simulink model "HANcoder_E407_TTA_Controller_v2"  (R2018b)
settings: Solver=FixedStepDiscrete  StartTime=0.0  StopTime=1  FixedStep=0.01  RelTol=1e-3
PreLoadFcn:
  | librarySetup
  | eval([bdroot,'_startup']) %Calling [modelName]_startup.m
values from neighbouring files (symbols this model uses):
  basic_cycle_duration_bc0 = TM_Reset_Board   + COMP_duration    (= 212)    [HANcoder_E407_TTA_Controller_v3_startup.m]
  basic_cycle_duration_bc1 = TM_Reset_Var_bc1 + COMP_duration    (= 288)    [HANcoder_E407_TTA_Controller_v3_startup.m]
  comm_delay_estimation1 = round(comm_delay_measured1*hardware_granularity/frequency_IRQ)    [HANcoder_E407_TTA_Controller_v3_startup.m]
  comm_delay_estimation2 = round(comm_delay_measured2*hardware_granularity/frequency_IRQ)    [HANcoder_E407_TTA_Controller_v3_startup.m]
  COMM_Period = 40    [HANcoder_E407_TTA_Controller_v3_startup.m]
  COMM_Phase1 = Simulink.Parameter    [HANcoder_E407_TTA_Controller_v3_startup.m]
  COMM_Phase2 = Simulink.Parameter    [HANcoder_E407_TTA_Controller_v3_startup.m]
  COMP_duration = 4    [HANcoder_E407_TTA_Controller_v3_startup.m]
  Controller1_Board = 1    [HANcoder_E407_TTA_Controller_v3_startup.m]
  Controller2_Board = 2    [HANcoder_E407_TTA_Controller_v3_startup.m]
  Controller3_Board = 3    [HANcoder_E407_TTA_Controller_v3_startup.m]
  delta_max = 1    [HANcoder_E407_TTA_Controller_v3_startup.m]
  delta_min = -1    [HANcoder_E407_TTA_Controller_v3_startup.m]
  delta_precision = 6    [HANcoder_E407_TTA_Controller_v3_startup.m]
  e_width = 0.1    [HANcoder_E407_TTA_Controller_v3_startup.m]
  frequency_IRQ = 100    [HANcoder_E407_TTA_Controller_v3_startup.m]
  HANtuneOverride = Simulink.Parameter    [HANcoder_E407_TTA_Controller_v3_startup.m]
  hardware_granularity = 1000000    [HANcoder_E407_TTA_Controller_v3_startup.m]
  I_a = 2.25    [HANcoder_E407_TTA_Controller_v3_startup.m]
  I_f = 2.25    [HANcoder_E407_TTA_Controller_v3_startup.m]
  idle_time_init = basic_cycle_duration_bc0 + basic_cycle_duration_bc1    (= 500)    [HANcoder_E407_TTA_Controller_v3_startup.m]
  Input_Gen_Board = 4    [HANcoder_E407_TTA_Controller_v3_startup.m]
  LA_Clock_Gr = 1    [HANcoder_E407_TTA_Controller_v3_startup.m]
  LA_COMM_Err = 1    [HANcoder_E407_TTA_Controller_v3_startup.m]
  LA_MEX_Flag = 1    [HANcoder_E407_TTA_Controller_v3_startup.m]
  LA_Task_Act = 1    [HANcoder_E407_TTA_Controller_v3_startup.m]
  m_v = 100.0    (= 100)    [HANcoder_E407_TTA_Controller_v3_startup.m]
  Master_Role = 1    [HANcoder_E407_TTA_Controller_v3_startup.m]
  matrix_cycle_duration = basic_cycle_duration_bc0 + basic_cycle_duration_bc1    (= 500)    [HANcoder_E407_TTA_Controller_v3_startup.m]
  matrix_rows = 2    [HANcoder_E407_TTA_Controller_v3_startup.m]
  max_num_msgs_CAN1 = 2^Tx_bit_number-1    (= 7)    [HANcoder_E407_TTA_Controller_v3_startup.m]
  max_num_msgs_CAN2 = max_num_msgs_CAN1    (= 7)    [HANcoder_E407_TTA_Controller_v3_startup.m]
  OutControl1_ID = 23    [HANcoder_E407_TTA_Controller_v3_startup.m]
  OutControl2_ID = 24    [HANcoder_E407_TTA_Controller_v3_startup.m]
  OutEmulator_ID = 25    [HANcoder_E407_TTA_Controller_v3_startup.m]
  R_al = 0.10    (= 0.1)    [HANcoder_E407_TTA_Controller_v3_startup.m]
  R_ar = 0.10    (= 0.1)    [HANcoder_E407_TTA_Controller_v3_startup.m]
  R_fl = 0.10    (= 0.1)    [HANcoder_E407_TTA_Controller_v3_startup.m]
  R_fr = 0.10    (= 0.1)    [HANcoder_E407_TTA_Controller_v3_startup.m]
  SensorValues_ID = 22    [HANcoder_E407_TTA_Controller_v3_startup.m]
  SetValues_ID = 21    [HANcoder_E407_TTA_Controller_v3_startup.m]
  Slave_Role = 2    [HANcoder_E407_TTA_Controller_v3_startup.m]
  speed_k_d = Simulink.Parameter    [HANcoder_E407_TTA_Controller_v3_startup.m]
  speed_k_i = Simulink.Parameter    [HANcoder_E407_TTA_Controller_v3_startup.m]
  speed_k_p = Simulink.Parameter    [HANcoder_E407_TTA_Controller_v3_startup.m]
  speed_max = 10    [HANcoder_E407_TTA_Controller_v3_startup.m]
  speed_min = -10    [HANcoder_E407_TTA_Controller_v3_startup.m]
  speed_precision = 3    [HANcoder_E407_TTA_Controller_v3_startup.m]
  Sync_ID = 1    [HANcoder_E407_TTA_Controller_v3_startup.m]
  tau_max = 5    [HANcoder_E407_TTA_Controller_v3_startup.m]
  tau_min = -5    [HANcoder_E407_TTA_Controller_v3_startup.m]
  tau_range = abs(tau_max) + abs(tau_min)    [HANcoder_E407_TTA_Controller_v3_startup.m]
  theta_max = (speed_max/R_fr)*matrix_cycle_duration*frequency_IRQ/hardware_granularity    (= 5)    [HANcoder_E407_TTA_Controller_v3_startup.m]
  theta_min = (-1)*theta_max    (= -5)    [HANcoder_E407_TTA_Controller_v3_startup.m]
  theta_precision = 7-(fix(log2(theta_max))+1)    [HANcoder_E407_TTA_Controller_v3_startup.m]
  Tl_a = 0.6    [HANcoder_E407_TTA_Controller_v3_startup.m]
  Tl_f = 0.6    [HANcoder_E407_TTA_Controller_v3_startup.m]
  TM_Check_Output_Control1 = TM_COMM_Output_Control1 + COMM_duration    (= 188)    [HANcoder_E407_TTA_Controller_v3_startup.m]
  TM_Check_Output_Control2 = TM_COMM_Output_Control2 + COMM_duration    (= 232)    [HANcoder_E407_TTA_Controller_v3_startup.m]
  TM_Check_Output_Emulator = TM_COMM_Output_Emulator + COMM_duration    (= 280)    [HANcoder_E407_TTA_Controller_v3_startup.m]
  TM_Check_Sensor_Values = TM_COMM_Sensor_Values + COMM_duration    (= 132)    [HANcoder_E407_TTA_Controller_v3_startup.m]
  TM_Check_Set_Values = TM_COMM_Set_Values + COMM_duration    (= 88)    [HANcoder_E407_TTA_Controller_v3_startup.m]
  TM_Check_Sync = TM_COMM_Sync   + COMM_duration    (= 40)    [HANcoder_E407_TTA_Controller_v3_startup.m]
  TM_Check_TOuts = TM_Count_Vote3 + COMP_duration    (= 196)    [HANcoder_E407_TTA_Controller_v3_startup.m]
  TM_Check_Vote1 = TM_COMM_Vote1  + COMM_duration    (= 92)    [HANcoder_E407_TTA_Controller_v3_startup.m]
  TM_Check_Vote2 = TM_COMM_Vote2  + COMM_duration    (= 140)    [HANcoder_E407_TTA_Controller_v3_startup.m]
  TM_Check_Vote3 = TM_COMM_Vote3  + COMM_duration    (= 188)    [HANcoder_E407_TTA_Controller_v3_startup.m]
  TM_COMM_Output_Control1 = TM_Velocity + COMP_duration    (= 148)    [HANcoder_E407_TTA_Controller_v3_startup.m]
  TM_COMM_Output_Control2 = TM_Check_Output_Control1 + COMP_duration    (= 192)    [HANcoder_E407_TTA_Controller_v3_startup.m]
  TM_COMM_Output_Emulator = TM_TMR + COMP_duration    (= 240)    [HANcoder_E407_TTA_Controller_v3_startup.m]
  TM_COMM_Sensor_Values = TM_Check_Set_Values + COMP_duration    (= 92)    [HANcoder_E407_TTA_Controller_v3_startup.m]
  TM_COMM_Set_Values = TM_Update_LT + COMP_duration    (= 48)    [HANcoder_E407_TTA_Controller_v3_startup.m]
  TM_COMM_Sync = basic_cycle_start    (= 0)    [HANcoder_E407_TTA_Controller_v3_startup.m]
  TM_COMM_Vote1 = TM_Vote_Dec    + COMP_duration    (= 52)    [HANcoder_E407_TTA_Controller_v3_startup.m]
  TM_COMM_Vote2 = TM_Count_Vote1 + COMP_duration    (= 100)    [HANcoder_E407_TTA_Controller_v3_startup.m]
  TM_COMM_Vote3 = TM_Count_Vote2 + COMP_duration    (= 148)    [HANcoder_E407_TTA_Controller_v3_startup.m]
  TM_Count_Vote1 = TM_Check_Vote1 + COMP_duration    (= 96)    [HANcoder_E407_TTA_Controller_v3_startup.m]
  TM_Count_Vote2 = TM_Check_Vote2 + COMP_duration    (= 144)    [HANcoder_E407_TTA_Controller_v3_startup.m]
  TM_Count_Vote3 = TM_Check_Vote3 + COMP_duration    (= 192)    [HANcoder_E407_TTA_Controller_v3_startup.m]
  TM_Data_bc0 = TM_COMM_Sync    (= 0)    [HANcoder_E407_TTA_Controller_v3_startup.m]
  TM_Data_bc1 = TM_Data_bc0(1:4)    [HANcoder_E407_TTA_Controller_v3_startup.m]
  TM_New_Master = TM_Check_TOuts + COMP_duration    (= 200)    [HANcoder_E407_TTA_Controller_v3_startup.m]
  TM_Reset_Board = TM_Reset_Var   + COMP_duration    (= 208)    [HANcoder_E407_TTA_Controller_v3_startup.m]
  TM_Reset_Var = TM_New_Master  + COMP_duration    (= 204)    [HANcoder_E407_TTA_Controller_v3_startup.m]
  TM_Reset_Var_bc1 = TM_Check_Output_Emulator + COMP_duration    (= 284)    [HANcoder_E407_TTA_Controller_v3_startup.m]
  TM_Steer = TM_Check_Sensor_Values + COMP_duration    (= 136)    [HANcoder_E407_TTA_Controller_v3_startup.m]
  TM_TMR = TM_Check_Output_Control2 + COMP_duration    (= 236)    [HANcoder_E407_TTA_Controller_v3_startup.m]
  TM_Torque = TM_Steer + COMP_duration    (= 140)    [HANcoder_E407_TTA_Controller_v3_startup.m]
  TM_Type_bc0 = COMM    (= 0)    [HANcoder_E407_TTA_Controller_v3_startup.m]
  TM_Type_bc1 = TM_Type_bc0(1:4)    [HANcoder_E407_TTA_Controller_v3_startup.m]
  TM_Update_LT = TM_Check_Sync  + COMP_duration    (= 44)    [HANcoder_E407_TTA_Controller_v3_startup.m]
  TM_Velocity = TM_Torque + COMP_duration    (= 144)    [HANcoder_E407_TTA_Controller_v3_startup.m]
  TM_Vote_Dec = TM_Update_LT   + COMP_duration    (= 48)    [HANcoder_E407_TTA_Controller_v3_startup.m]
  torque_a_k_d = Simulink.Parameter    [HANcoder_E407_TTA_Controller_v3_startup.m]
  torque_a_k_i = Simulink.Parameter    [HANcoder_E407_TTA_Controller_v3_startup.m]
  torque_a_k_p = Simulink.Parameter    [HANcoder_E407_TTA_Controller_v3_startup.m]
  torque_f_k_d = Simulink.Parameter    [HANcoder_E407_TTA_Controller_v3_startup.m]
  torque_f_k_i = Simulink.Parameter    [HANcoder_E407_TTA_Controller_v3_startup.m]
  torque_f_k_p = Simulink.Parameter    [HANcoder_E407_TTA_Controller_v3_startup.m]
  torque_precision = 4    [HANcoder_E407_TTA_Controller_v3_startup.m]
  Vehicle_Em_Board = 5    [HANcoder_E407_TTA_Controller_v3_startup.m]
  Vote1_ID = 11    [HANcoder_E407_TTA_Controller_v3_startup.m]
  Vote2_ID = 12    [HANcoder_E407_TTA_Controller_v3_startup.m]
  Vote3_ID = 13    [HANcoder_E407_TTA_Controller_v3_startup.m]
undefined symbols (not defined in the file or in its folder): A0, A1, A2, A3, A4, CON2
libraries: hdlsllib x235, HANcoder_STM32_Target x25, simulink x3, simulink_extras x1
(part 21 of 22)

== system HANcoder_E407_TTA_Controller_v2/HANcoder STM32 Target - E407-STM32 algorithm/Global Ticks Increment/CAN Management/Matrix Cycle Manager/Subsystem/controller basic cycle 1/COMP Task - Rx_Output_Control2_Check/Process_Messages/Demux message CAN1 and check coherence1/msg_count>2_DEBUG ==
  note: If this board received during this COMM a message
      | with a count greater than 1, it means the first message
      | sent was missed, but at least one later msg reached
      | this board.
  msg_c : Inport
  Constant : Constant
  Constant1 : Constant
  Data Store Read : DataStoreRead  DataStoreName=msg_count_DEBUG
  Data Store Read1 : DataStoreRead  DataStoreName=msg_count_DEBUG
  Data Store Write : DataStoreWrite  DataStoreName=msg_count_DEBUG
  GreaterThan : RelationalOperator  Operator=>  OutDataTypeStr=boolean  RndMeth=Simplest
  Plus : Sum
  Switch : Switch  Criteria=u2 > Threshold
  wires:
  msg_c/1 -> GreaterThan/1
  Data Store Read/1 -> Switch/3
  Plus/1 -> Switch/1
  Data Store Read1/1 -> Plus/1
  Constant/1 -> Plus/2
  Switch/1 -> Data Store Write/1
  GreaterThan/1 -> Switch/2
  Constant1/1 -> GreaterThan/2

== system HANcoder_E407_TTA_Controller_v2/HANcoder STM32 Target - E407-STM32 algorithm/Global Ticks Increment/CAN Management/Matrix Cycle Manager/Subsystem/controller basic cycle 1/COMP Task - Rx_Output_Emulator_Check/Process_Messages/Demux message CAN1 and check coherence/Subsystem ==
  Msg_Temporal_Data : Inport
  Bit Shift : hdlsllib/Logic and Bit Operations/Bit Shift  mode=Shift Right Logical  N=7
      settings: SourceProductName=HDL Coder  SourceProductBaseCode=HD
  Bit Shift1 : hdlsllib/Logic and Bit Operations/Bit Shift  mode=Shift Right Logical  N=5
      settings: SourceProductName=HDL Coder  SourceProductBaseCode=HD
  Bit Shift2 : hdlsllib/Logic and Bit Operations/Bit Shift  mode=Shift Right Logical  N=4
      settings: SourceProductName=HDL Coder  SourceProductBaseCode=HD
  Bit Shift3 : hdlsllib/Logic and Bit Operations/Bit Shift  mode=Shift Left Logical  N=1
      settings: SourceProductName=HDL Coder  SourceProductBaseCode=HD
  Bit Shift4 : hdlsllib/Logic and Bit Operations/Bit Shift  mode=Shift Left Logical  N=4
      settings: SourceProductName=HDL Coder  SourceProductBaseCode=HD
  basic_cycle : Outport
  msg_count : Outport  Port=2
  board_id : Outport  Port=3
  wires:
  Bit Shift2/1 -> board_id/1
  Bit Shift/1 -> basic_cycle/1
  Msg_Temporal_Data/1 -> Bit Shift3/1, Bit Shift/1, Bit Shift4/1
  Bit Shift3/1 -> Bit Shift1/1
  Bit Shift1/1 -> msg_count/1
  Bit Shift4/1 -> Bit Shift2/1

== system HANcoder_E407_TTA_Controller_v2/HANcoder STM32 Target - E407-STM32 algorithm/Global Ticks Increment/CAN Management/Matrix Cycle Manager/Subsystem/controller basic cycle 1/COMP Task - Rx_Output_Emulator_Check/Process_Messages/Demux message CAN1 and check coherence/msg_count>2_DEBUG ==
  note: If this board received during this COMM a message
      | with a count greater than 1, it means the first message
      | sent was missed, but at least one later msg reached
      | this board.
  msg_c : Inport
  Constant : Constant
  Constant1 : Constant
  Data Store Read : DataStoreRead  DataStoreName=msg_count_DEBUG
  Data Store Read1 : DataStoreRead  DataStoreName=msg_count_DEBUG
  Data Store Write : DataStoreWrite  DataStoreName=msg_count_DEBUG
  GreaterThan : RelationalOperator  Operator=>  OutDataTypeStr=boolean  RndMeth=Simplest
  Plus : Sum
  Switch : Switch  Criteria=u2 > Threshold
  wires:
  Constant1/1 -> GreaterThan/2
  GreaterThan/1 -> Switch/2
  Switch/1 -> Data Store Write/1
  Constant/1 -> Plus/2
  Data Store Read1/1 -> Plus/1
  Plus/1 -> Switch/1
  Data Store Read/1 -> Switch/3
  msg_c/1 -> GreaterThan/1

== system HANcoder_E407_TTA_Controller_v2/HANcoder STM32 Target - E407-STM32 algorithm/Global Ticks Increment/CAN Management/Matrix Cycle Manager/Subsystem/controller basic cycle 1/COMP Task - Rx_Output_Emulator_Check/Process_Messages/Demux message CAN1 and check coherence1/Subsystem ==
  Msg_Temporal_Data : Inport
  Bit Shift : hdlsllib/Logic and Bit Operations/Bit Shift  mode=Shift Right Logical  N=7
      settings: SourceProductName=HDL Coder  SourceProductBaseCode=HD
  Bit Shift1 : hdlsllib/Logic and Bit Operations/Bit Shift  mode=Shift Right Logical  N=5
      settings: SourceProductName=HDL Coder  SourceProductBaseCode=HD
  Bit Shift2 : hdlsllib/Logic and Bit Operations/Bit Shift  mode=Shift Right Logical  N=4
      settings: SourceProductName=HDL Coder  SourceProductBaseCode=HD
  Bit Shift3 : hdlsllib/Logic and Bit Operations/Bit Shift  mode=Shift Left Logical  N=1
      settings: SourceProductName=HDL Coder  SourceProductBaseCode=HD
  Bit Shift4 : hdlsllib/Logic and Bit Operations/Bit Shift  mode=Shift Left Logical  N=4
      settings: SourceProductName=HDL Coder  SourceProductBaseCode=HD
  basic_cycle : Outport
  msg_count : Outport  Port=2
  board_id : Outport  Port=3
  wires:
  Bit Shift4/1 -> Bit Shift2/1
  Bit Shift3/1 -> Bit Shift1/1
  Bit Shift2/1 -> board_id/1
  Bit Shift1/1 -> msg_count/1
  Msg_Temporal_Data/1 -> Bit Shift3/1, Bit Shift/1, Bit Shift4/1
  Bit Shift/1 -> basic_cycle/1

== system HANcoder_E407_TTA_Controller_v2/HANcoder STM32 Target - E407-STM32 algorithm/Global Ticks Increment/CAN Management/Matrix Cycle Manager/Subsystem/controller basic cycle 1/COMP Task - Rx_Output_Emulator_Check/Process_Messages/Demux message CAN1 and check coherence1/msg_count>2_DEBUG ==
  note: If this board received during this COMM a message
      | with a count greater than 1, it means the first message
      | sent was missed, but at least one later msg reached
      | this board.
  msg_c : Inport
  Constant : Constant
  Constant1 : Constant
  Data Store Read : DataStoreRead  DataStoreName=msg_count_DEBUG
  Data Store Read1 : DataStoreRead  DataStoreName=msg_count_DEBUG
  Data Store Write : DataStoreWrite  DataStoreName=msg_count_DEBUG
  GreaterThan : RelationalOperator  Operator=>  OutDataTypeStr=boolean  RndMeth=Simplest
  Plus : Sum
  Switch : Switch  Criteria=u2 > Threshold
  wires:
  Constant1/1 -> GreaterThan/2
  GreaterThan/1 -> Switch/2
  Switch/1 -> Data Store Write/1
  Constant/1 -> Plus/2
  Data Store Read1/1 -> Plus/1
  Plus/1 -> Switch/1
  Data Store Read/1 -> Switch/3
  msg_c/1 -> GreaterThan/1

== system HANcoder_E407_TTA_Controller_v2/HANcoder STM32 Target - E407-STM32 algorithm/Global Ticks Increment/CAN Management/Matrix Cycle Manager/Subsystem/controller basic cycle 1/COMP Task - Rx_Sensor_Values_Check/Process_Messages/Demux message CAN1 and check coherence/Subsystem ==
  Msg_Temporal_Data : Inport
  Bit Shift : hdlsllib/Logic and Bit Operations/Bit Shift  mode=Shift Right Logical  N=7
      settings: SourceProductName=HDL Coder  SourceProductBaseCode=HD
  Bit Shift1 : hdlsllib/Logic and Bit Operations/Bit Shift  mode=Shift Right Logical  N=5
      settings: SourceProductName=HDL Coder  SourceProductBaseCode=HD
  Bit Shift2 : hdlsllib/Logic and Bit Operations/Bit Shift  mode=Shift Right Logical  N=4
      settings: SourceProductName=HDL Coder  SourceProductBaseCode=HD
  Bit Shift3 : hdlsllib/Logic and Bit Operations/Bit Shift  mode=Shift Left Logical  N=1
      settings: SourceProductName=HDL Coder  SourceProductBaseCode=HD
  Bit Shift4 : hdlsllib/Logic and Bit Operations/Bit Shift  mode=Shift Left Logical  N=4
      settings: SourceProductName=HDL Coder  SourceProductBaseCode=HD
  basic_cycle : Outport
  msg_count : Outport  Port=2
  board_id : Outport  Port=3
  wires:
  Bit Shift4/1 -> Bit Shift2/1
  Bit Shift1/1 -> msg_count/1
  Bit Shift3/1 -> Bit Shift1/1
  Msg_Temporal_Data/1 -> Bit Shift4/1, Bit Shift/1, Bit Shift3/1
  Bit Shift/1 -> basic_cycle/1
  Bit Shift2/1 -> board_id/1

== system HANcoder_E407_TTA_Controller_v2/HANcoder STM32 Target - E407-STM32 algorithm/Global Ticks Increment/CAN Management/Matrix Cycle Manager/Subsystem/controller basic cycle 1/COMP Task - Rx_Sensor_Values_Check/Process_Messages/Demux message CAN1 and check coherence/msg_count>2_DEBUG ==
  note: If this board received during this COMM a message
      | with a count greater than 1, it means the first message
      | sent was missed, but at least one later msg reached
      | this board.
  msg_c : Inport
  Constant : Constant
  Constant1 : Constant
  Data Store Read : DataStoreRead  DataStoreName=msg_count_DEBUG
  Data Store Read1 : DataStoreRead  DataStoreName=msg_count_DEBUG
  Data Store Write : DataStoreWrite  DataStoreName=msg_count_DEBUG
  GreaterThan : RelationalOperator  Operator=>  OutDataTypeStr=boolean  RndMeth=Simplest
  Plus : Sum
  Switch : Switch  Criteria=u2 > Threshold
  wires:
  msg_c/1 -> GreaterThan/1
  Data Store Read/1 -> Switch/3
  Plus/1 -> Switch/1
  Data Store Read1/1 -> Plus/1
  Constant/1 -> Plus/2
  Switch/1 -> Data Store Write/1
  GreaterThan/1 -> Switch/2
  Constant1/1 -> GreaterThan/2

== system HANcoder_E407_TTA_Controller_v2/HANcoder STM32 Target - E407-STM32 algorithm/Global Ticks Increment/CAN Management/Matrix Cycle Manager/Subsystem/controller basic cycle 1/COMP Task - Rx_Sensor_Values_Check/Process_Messages/Demux message CAN1 and check coherence1/Subsystem ==
  Msg_Temporal_Data : Inport
  Bit Shift : hdlsllib/Logic and Bit Operations/Bit Shift  mode=Shift Right Logical  N=7
      settings: SourceProductName=HDL Coder  SourceProductBaseCode=HD
  Bit Shift1 : hdlsllib/Logic and Bit Operations/Bit Shift  mode=Shift Right Logical  N=5
      settings: SourceProductName=HDL Coder  SourceProductBaseCode=HD
  Bit Shift2 : hdlsllib/Logic and Bit Operations/Bit Shift  mode=Shift Right Logical  N=4
      settings: SourceProductName=HDL Coder  SourceProductBaseCode=HD
  Bit Shift3 : hdlsllib/Logic and Bit Operations/Bit Shift  mode=Shift Left Logical  N=1
      settings: SourceProductName=HDL Coder  SourceProductBaseCode=HD
  Bit Shift4 : hdlsllib/Logic and Bit Operations/Bit Shift  mode=Shift Left Logical  N=4
      settings: SourceProductName=HDL Coder  SourceProductBaseCode=HD
  basic_cycle : Outport
  msg_count : Outport  Port=2
  board_id : Outport  Port=3
  wires:
  Bit Shift/1 -> basic_cycle/1
  Msg_Temporal_Data/1 -> Bit Shift4/1, Bit Shift/1, Bit Shift3/1
  Bit Shift1/1 -> msg_count/1
  Bit Shift2/1 -> board_id/1
  Bit Shift3/1 -> Bit Shift1/1
  Bit Shift4/1 -> Bit Shift2/1

== system HANcoder_E407_TTA_Controller_v2/HANcoder STM32 Target - E407-STM32 algorithm/Global Ticks Increment/CAN Management/Matrix Cycle Manager/Subsystem/controller basic cycle 1/COMP Task - Rx_Sensor_Values_Check/Process_Messages/Demux message CAN1 and check coherence1/msg_count>2_DEBUG ==
  note: If this board received during this COMM a message
      | with a count greater than 1, it means the first message
      | sent was missed, but at least one later msg reached
      | this board.
  msg_c : Inport
  Constant : Constant
  Constant1 : Constant
  Data Store Read : DataStoreRead  DataStoreName=msg_count_DEBUG
  Data Store Read1 : DataStoreRead  DataStoreName=msg_count_DEBUG
  Data Store Write : DataStoreWrite  DataStoreName=msg_count_DEBUG
  GreaterThan : RelationalOperator  Operator=>  OutDataTypeStr=boolean  RndMeth=Simplest
  Plus : Sum
  Switch : Switch  Criteria=u2 > Threshold
  wires:
  msg_c/1 -> GreaterThan/1
  Data Store Read/1 -> Switch/3
  Plus/1 -> Switch/1
  Data Store Read1/1 -> Plus/1
  Constant/1 -> Plus/2
  Switch/1 -> Data Store Write/1
  GreaterThan/1 -> Switch/2
  Constant1/1 -> GreaterThan/2

== system HANcoder_E407_TTA_Controller_v2/HANcoder STM32 Target - E407-STM32 algorithm/Global Ticks Increment/CAN Management/Matrix Cycle Manager/Subsystem/controller basic cycle 1/COMP Task - Rx_Sensor_Values_Check/Update Msg buffer/Sensor Values Rx Update/Inputs Rx OK ==
  note: Matrix cycles since last input value
  note: Ticks to seconds conversion
  note: For derivatives and integrals it is important to keep
      | track of how much time has passed since the last
      | time we received a set or sensor value.
  Enable : EnablePort
  Constant : Constant  Value=matrix_cycle_duration
  Constant1 : Constant
  Data Store Read : DataStoreRead  DataStoreName=mc_counter
  Data Store Write : DataStoreWrite  Priority=1  DataStoreName=rx_data_incr_time
  Data Store Write1 : DataStoreWrite  Priority=2  DataStoreName=mc_counter
  Gain : Gain  Gain=frequency_IRQ/hardware_granularity
  Multiply : Product
  wires:
  Constant/1 -> Gain/1
  Gain/1 -> Multiply/1
  Data Store Read/1 -> Multiply/2
  Multiply/1 -> Data Store Write/1
  Constant1/1 -> Data Store Write1/1

== system HANcoder_E407_TTA_Controller_v2/HANcoder STM32 Target - E407-STM32 algorithm/Global Ticks Increment/CAN Management/Matrix Cycle Manager/Subsystem/controller basic cycle 1/COMP Task - Rx_Sensor_Values_Check/Update Msg buffer/Sensor Values Rx Update/Not enough inputs ==
  note: If no inputs received, no calculations are done.
      | Next time set and sensor values are received
      | it is important to keep track of how much time
      | has passed for derivatives and integrals.
  Enable : EnablePort
  Constant : Constant
  Data Store Read : DataStoreRead  DataStoreName=mc_counter
  Data Store Write1 : DataStoreWrite  DataStoreName=mc_counter
  Minus : Sum
  wires:
  Data Store Read/1 -> Minus/1
  Constant/1 -> Minus/2
  Minus/1 -> Data Store Write1/1

== system HANcoder_E407_TTA_Controller_v2/HANcoder STM32 Target - E407-STM32 algorithm/Global Ticks Increment/CAN Management/Matrix Cycle Manager/Subsystem/controller basic cycle 1/COMP Task - Rx_Sensor_Values_Check/Update Msg buffer/Sensor Values Rx Update/uint8_2float ==
  precision : Inport
  value : Inport  Port=2
  Bit Shift : hdlsllib/Logic and Bit Operations/Bit Shift  mode=Shift Right Logical  N=7
      settings: SourceProductName=HDL Coder  SourceProductBaseCode=HD
  Bit Shift1 : hdlsllib/Logic and Bit Operations/Bit Shift  mode=Shift Left Logical  N=7
      settings: SourceProductName=HDL Coder  SourceProductBaseCode=HD
  Cast1 : DataTypeConversion  OutDataTypeStr=double
  Constant1 : Constant  Value=2
  Constant2 : Constant  Value=2
  Divide : Product  Inputs=*/
  Fix1 : Rounding  Operator=fix
  Gain : Gain  Gain=-1
  Gain1 : Gain  Gain=-1
  Minus : Sum  Inputs=-+
  Minus1 : Sum  Inputs=+-
  Minus2 : Sum
  Multiply : Product
  Multiply1 : Product
  Power : Math  Priority=5  Operator=pow  SaturateOnIntegerOverflow=on
  Power1 : Math  Priority=5  Operator=pow  SaturateOnIntegerOverflow=on
  Switch : Switch  Criteria=u2 > Threshold
  decoded : Outport
  wires:
  Bit Shift/1 -> Bit Shift1/1, Switch/2
  value/1 -> Cast1/1, Bit Shift/1
  Minus/1 -> Divide/1, Minus1/1
  Fix1/1 -> Minus2/2, Multiply1/1
  Multiply1/1 -> Minus1/2
  Minus1/1 -> Multiply/1
  Constant1/1 -> Power/1
  Gain/1 -> Power/2
  Power/1 -> Multiply/2
  [precision] -> Gain/1
  Multiply/1 -> Minus2/1
  Minus2/1 -> Gain1/1, Switch/3
  Gain1/1 -> Switch/1
  Switch/1 -> decoded/1
  Divide/1 -> Fix1/1
  Cast1/1 -> Minus/2
  precision/1 -> Power1/2, [precision]
  Constant2/1 -> Power1/1
  Power1/1 -> [prec_pow]
  [prec_pow] -> Divide/2
  [prec_pow] -> Multiply1/2
  Bit Shift1/1 -> Minus/1

== system HANcoder_E407_TTA_Controller_v2/HANcoder STM32 Target - E407-STM32 algorithm/Global Ticks Increment/CAN Management/Matrix Cycle Manager/Subsystem/controller basic cycle 1/COMP Task - Rx_Sensor_Values_Check/Update Msg buffer/Sensor Values Rx Update/uint8_2float1 ==
  precision : Inport
  value : Inport  Port=2
  Bit Shift : hdlsllib/Logic and Bit Operations/Bit Shift  mode=Shift Right Logical  N=7
      settings: SourceProductName=HDL Coder  SourceProductBaseCode=HD
  Bit Shift1 : hdlsllib/Logic and Bit Operations/Bit Shift  mode=Shift Left Logical  N=7
      settings: SourceProductName=HDL Coder  SourceProductBaseCode=HD
  Cast1 : DataTypeConversion  OutDataTypeStr=double
  Constant1 : Constant  Value=2
  Constant2 : Constant  Value=2
  Divide : Product  Inputs=*/
  Fix1 : Rounding  Operator=fix
  Gain : Gain  Gain=-1
  Gain1 : Gain  Gain=-1
  Minus : Sum  Inputs=-+
  Minus1 : Sum  Inputs=+-
  Minus2 : Sum
  Multiply : Product
  Multiply1 : Product
  Power : Math  Priority=5  Operator=pow  SaturateOnIntegerOverflow=on
  Power1 : Math  Priority=5  Operator=pow  SaturateOnIntegerOverflow=on
  Switch : Switch  Criteria=u2 > Threshold
  decoded : Outport
  wires:
  Bit Shift1/1 -> Minus/1
  [prec_pow] -> Multiply1/2
  [prec_pow] -> Divide/2
  Power1/1 -> [prec_pow]
  Constant2/1 -> Power1/1
  precision/1 -> [precision], Power1/2
  Cast1/1 -> Minus/2
  Divide/1 -> Fix1/1
  Switch/1 -> decoded/1
  Gain1/1 -> Switch/1
  Minus2/1 -> Switch/3, Gain1/1
  Multiply/1 -> Minus2/1
  [precision] -> Gain/1
  Power/1 -> Multiply/2
  Gain/1 -> Power/2
  Constant1/1 -> Power/1
  Minus1/1 -> Multiply/1
  Multiply1/1 -> Minus1/2
  Fix1/1 -> Multiply1/1, Minus2/2
  Minus/1 -> Minus1/1, Divide/1
  value/1 -> Bit Shift/1, Cast1/1
  Bit Shift/1 -> Switch/2, Bit Shift1/1

== system HANcoder_E407_TTA_Controller_v2/HANcoder STM32 Target - E407-STM32 algorithm/Global Ticks Increment/CAN Management/Matrix Cycle Manager/Subsystem/controller basic cycle 1/COMP Task - Rx_Sensor_Values_Check/Update Msg buffer/Sensor Values Rx Update/uint8_2float2 ==
  precision : Inport
  value : Inport  Port=2
  Bit Shift : hdlsllib/Logic and Bit Operations/Bit Shift  mode=Shift Right Logical  N=7
      settings: SourceProductName=HDL Coder  SourceProductBaseCode=HD
  Bit Shift1 : hdlsllib/Logic and Bit Operations/Bit Shift  mode=Shift Left Logical  N=7
      settings: SourceProductName=HDL Coder  SourceProductBaseCode=HD
  Cast1 : DataTypeConversion  OutDataTypeStr=double
  Constant1 : Constant  Value=2
  Constant2 : Constant  Value=2
  Divide : Product  Inputs=*/
  Fix1 : Rounding  Operator=fix
  Gain : Gain  Gain=-1
  Gain1 : Gain  Gain=-1
  Minus : Sum  Inputs=-+
  Minus1 : Sum  Inputs=+-
  Minus2 : Sum
  Multiply : Product
  Multiply1 : Product
  Power : Math  Priority=5  Operator=pow  SaturateOnIntegerOverflow=on
  Power1 : Math  Priority=5  Operator=pow  SaturateOnIntegerOverflow=on
  Switch : Switch  Criteria=u2 > Threshold
  decoded : Outport
  wires:
  Bit Shift/1 -> Bit Shift1/1, Switch/2
  value/1 -> Cast1/1, Bit Shift/1
  Minus/1 -> Divide/1, Minus1/1
  Fix1/1 -> Minus2/2, Multiply1/1
  Multiply1/1 -> Minus1/2
  Minus1/1 -> Multiply/1
  Constant1/1 -> Power/1
  Gain/1 -> Power/2
  Power/1 -> Multiply/2
  [precision] -> Gain/1
  Multiply/1 -> Minus2/1
  Minus2/1 -> Gain1/1, Switch/3
  Gain1/1 -> Switch/1
  Switch/1 -> decoded/1
  Divide/1 -> Fix1/1
  Cast1/1 -> Minus/2
  precision/1 -> Power1/2, [precision]
  Constant2/1 -> Power1/1
  Power1/1 -> [prec_pow]
  [prec_pow] -> Divide/2
  [prec_pow] -> Multiply1/2
  Bit Shift1/1 -> Minus/1

== system HANcoder_E407_TTA_Controller_v2/HANcoder STM32 Target - E407-STM32 algorithm/Global Ticks Increment/CAN Management/Matrix Cycle Manager/Subsystem/controller basic cycle 1/COMP Task - Rx_Sensor_Values_Check/Update Msg buffer/Sensor Values Rx Update/uint8_2float3 ==
  precision : Inport
  value : Inport  Port=2
  Bit Shift : hdlsllib/Logic and Bit Operations/Bit Shift  mode=Shift Right Logical  N=7
      settings: SourceProductName=HDL Coder  SourceProductBaseCode=HD
  Bit Shift1 : hdlsllib/Logic and Bit Operations/Bit Shift  mode=Shift Left Logical  N=7
      settings: SourceProductName=HDL Coder  SourceProductBaseCode=HD
  Cast1 : DataTypeConversion  OutDataTypeStr=double
  Constant1 : Constant  Value=2
  Constant2 : Constant  Value=2
  Divide : Product  Inputs=*/
  Fix1 : Rounding  Operator=fix
  Gain : Gain  Gain=-1
  Gain1 : Gain  Gain=-1
  Minus : Sum  Inputs=-+
  Minus1 : Sum  Inputs=+-
  Minus2 : Sum
  Multiply : Product
  Multiply1 : Product
  Power : Math  Priority=5  Operator=pow  SaturateOnIntegerOverflow=on
  Power1 : Math  Priority=5  Operator=pow  SaturateOnIntegerOverflow=on
  Switch : Switch  Criteria=u2 > Threshold
  decoded : Outport
  wires:
  Bit Shift1/1 -> Minus/1
  [prec_pow] -> Multiply1/2
  [prec_pow] -> Divide/2
  Power1/1 -> [prec_pow]
  Constant2/1 -> Power1/1
  precision/1 -> [precision], Power1/2
  Cast1/1 -> Minus/2
  Divide/1 -> Fix1/1
  Switch/1 -> decoded/1
  Gain1/1 -> Switch/1
  Minus2/1 -> Switch/3, Gain1/1
  Multiply/1 -> Minus2/1
  [precision] -> Gain/1
  Power/1 -> Multiply/2
  Gain/1 -> Power/2
  Constant1/1 -> Power/1
  Minus1/1 -> Multiply/1
  Multiply1/1 -> Minus1/2
  Fix1/1 -> Multiply1/1, Minus2/2
  Minus/1 -> Minus1/1, Divide/1
  value/1 -> Bit Shift/1, Cast1/1
  Bit Shift/1 -> Switch/2, Bit Shift1/1

== system HANcoder_E407_TTA_Controller_v2/HANcoder STM32 Target - E407-STM32 algorithm/Global Ticks Increment/CAN Management/Matrix Cycle Manager/Subsystem/controller basic cycle 1/COMP Task - Rx_Set_Values_Check/Process_Messages/Demux message CAN1 and check coherence/Subsystem ==
  Msg_Temporal_Data : Inport
  Bit Shift : hdlsllib/Logic and Bit Operations/Bit Shift  mode=Shift Right Logical  N=7
      settings: SourceProductName=HDL Coder  SourceProductBaseCode=HD
  Bit Shift1 : hdlsllib/Logic and Bit Operations/Bit Shift  mode=Shift Right Logical  N=5
      settings: SourceProductName=HDL Coder  SourceProductBaseCode=HD
  Bit Shift2 : hdlsllib/Logic and Bit Operations/Bit Shift  mode=Shift Right Logical  N=4
      settings: SourceProductName=HDL Coder  SourceProductBaseCode=HD
  Bit Shift3 : hdlsllib/Logic and Bit Operations/Bit Shift  mode=Shift Left Logical  N=1
      settings: SourceProductName=HDL Coder  SourceProductBaseCode=HD
  Bit Shift4 : hdlsllib/Logic and Bit Operations/Bit Shift  mode=Shift Left Logical  N=4
      settings: SourceProductName=HDL Coder  SourceProductBaseCode=HD
  basic_cycle : Outport
  msg_count : Outport  Port=2
  board_id : Outport  Port=3
  wires:
  Bit Shift2/1 -> board_id/1
  Bit Shift/1 -> basic_cycle/1
  Msg_Temporal_Data/1 -> Bit Shift3/1, Bit Shift/1, Bit Shift4/1
  Bit Shift3/1 -> Bit Shift1/1
  Bit Shift1/1 -> msg_count/1
  Bit Shift4/1 -> Bit Shift2/1

== system HANcoder_E407_TTA_Controller_v2/HANcoder STM32 Target - E407-STM32 algorithm/Global Ticks Increment/CAN Management/Matrix Cycle Manager/Subsystem/controller basic cycle 1/COMP Task - Rx_Set_Values_Check/Process_Messages/Demux message CAN1 and check coherence/msg_count>2_DEBUG ==
  note: If this board received during this COMM a message
      | with a count greater than 1, it means the first message
      | sent was missed, but at least one later msg reached
      | this board.
  msg_c : Inport
  Constant : Constant
  Constant1 : Constant
  Data Store Read : DataStoreRead  DataStoreName=msg_count_DEBUG
  Data Store Read1 : DataStoreRead  DataStoreName=msg_count_DEBUG
  Data Store Write : DataStoreWrite  DataStoreName=msg_count_DEBUG
  GreaterThan : RelationalOperator  Operator=>  OutDataTypeStr=boolean  RndMeth=Simplest
  Plus : Sum
  Switch : Switch  Criteria=u2 > Threshold
  wires:
  Constant1/1 -> GreaterThan/2
  GreaterThan/1 -> Switch/2
  Switch/1 -> Data Store Write/1
  Constant/1 -> Plus/2
  Data Store Read1/1 -> Plus/1
  Plus/1 -> Switch/1
  Data Store Read/1 -> Switch/3
  msg_c/1 -> GreaterThan/1

== system HANcoder_E407_TTA_Controller_v2/HANcoder STM32 Target - E407-STM32 algorithm/Global Ticks Increment/CAN Management/Matrix Cycle Manager/Subsystem/controller basic cycle 1/COMP Task - Rx_Set_Values_Check/Process_Messages/Demux message CAN1 and check coherence1/Subsystem ==
  Msg_Temporal_Data : Inport
  Bit Shift : hdlsllib/Logic and Bit Operations/Bit Shift  mode=Shift Right Logical  N=7
      settings: SourceProductName=HDL Coder  SourceProductBaseCode=HD
  Bit Shift1 : hdlsllib/Logic and Bit Operations/Bit Shift  mode=Shift Right Logical  N=5
      settings: SourceProductName=HDL Coder  SourceProductBaseCode=HD
  Bit Shift2 : hdlsllib/Logic and Bit Operations/Bit Shift  mode=Shift Right Logical  N=4
      settings: SourceProductName=HDL Coder  SourceProductBaseCode=HD
  Bit Shift3 : hdlsllib/Logic and Bit Operations/Bit Shift  mode=Shift Left Logical  N=1
      settings: SourceProductName=HDL Coder  SourceProductBaseCode=HD
  Bit Shift4 : hdlsllib/Logic and Bit Operations/Bit Shift  mode=Shift Left Logical  N=4
      settings: SourceProductName=HDL Coder  SourceProductBaseCode=HD
  basic_cycle : Outport
  msg_count : Outport  Port=2
  board_id : Outport  Port=3
  wires:
  Bit Shift4/1 -> Bit Shift2/1
  Bit Shift3/1 -> Bit Shift1/1
  Bit Shift2/1 -> board_id/1
  Bit Shift1/1 -> msg_count/1
  Msg_Temporal_Data/1 -> Bit Shift3/1, Bit Shift/1, Bit Shift4/1
  Bit Shift/1 -> basic_cycle/1

== system HANcoder_E407_TTA_Controller_v2/HANcoder STM32 Target - E407-STM32 algorithm/Global Ticks Increment/CAN Management/Matrix Cycle Manager/Subsystem/controller basic cycle 1/COMP Task - Rx_Set_Values_Check/Process_Messages/Demux message CAN1 and check coherence1/msg_count>2_DEBUG ==
  note: If this board received during this COMM a message
      | with a count greater than 1, it means the first message
      | sent was missed, but at least one later msg reached
      | this board.
  msg_c : Inport
  Constant : Constant
  Constant1 : Constant
  Data Store Read : DataStoreRead  DataStoreName=msg_count_DEBUG
  Data Store Read1 : DataStoreRead  DataStoreName=msg_count_DEBUG
  Data Store Write : DataStoreWrite  DataStoreName=msg_count_DEBUG
  GreaterThan : RelationalOperator  Operator=>  OutDataTypeStr=boolean  RndMeth=Simplest
  Plus : Sum
  Switch : Switch  Criteria=u2 > Threshold
  wires:
  Constant1/1 -> GreaterThan/2
  GreaterThan/1 -> Switch/2
  Switch/1 -> Data Store Write/1
  Constant/1 -> Plus/2
  Data Store Read1/1 -> Plus/1
  Plus/1 -> Switch/1
  Data Store Read/1 -> Switch/3
  msg_c/1 -> GreaterThan/1

== system HANcoder_E407_TTA_Controller_v2/HANcoder STM32 Target - E407-STM32 algorithm/Global Ticks Increment/CAN Management/Matrix Cycle Manager/Subsystem/controller basic cycle 1/COMP Task - Rx_Set_Values_Check/Update Msg buffer/Set Values Update/uint8_2float ==
  precision : Inport
  value : Inport  Port=2
  Bit Shift : hdlsllib/Logic and Bit Operations/Bit Shift  mode=Shift Right Logical  N=7
      settings: SourceProductName=HDL Coder  SourceProductBaseCode=HD
  Bit Shift1 : hdlsllib/Logic and Bit Operations/Bit Shift  mode=Shift Left Logical  N=7
      settings: SourceProductName=HDL Coder  SourceProductBaseCode=HD
  Cast1 : DataTypeConversion  OutDataTypeStr=double
  Constant1 : Constant  Value=2
  Constant2 : Constant  Value=2
  Divide : Product  Inputs=*/
  Fix1 : Rounding  Operator=fix
  Gain : Gain  Gain=-1
  Gain1 : Gain  Gain=-1
  Minus : Sum  Inputs=-+
  Minus1 : Sum  Inputs=+-
  Minus2 : Sum
  Multiply : Product
  Multiply1 : Product
  Power : Math  Priority=5  Operator=pow  SaturateOnIntegerOverflow=on
  Power1 : Math  Priority=5  Operator=pow  SaturateOnIntegerOverflow=on
  Switch : Switch  Criteria=u2 > Threshold
  decoded : Outport
  wires:
  Bit Shift/1 -> Bit Shift1/1, Switch/2
  value/1 -> Cast1/1, Bit Shift/1
  Minus/1 -> Divide/1, Minus1/1
  Fix1/1 -> Minus2/2, Multiply1/1
  Multiply1/1 -> Minus1/2
  Minus1/1 -> Multiply/1
  Constant1/1 -> Power/1
  Gain/1 -> Power/2
  Power/1 -> Multiply/2
  [precision] -> Gain/1
  Multiply/1 -> Minus2/1
  Minus2/1 -> Gain1/1, Switch/3
  Gain1/1 -> Switch/1
  Switch/1 -> decoded/1
  Divide/1 -> Fix1/1
  Cast1/1 -> Minus/2
  precision/1 -> Power1/2, [precision]
  Constant2/1 -> Power1/1
  Power1/1 -> [prec_pow]
  [prec_pow] -> Divide/2
  [prec_pow] -> Multiply1/2
  Bit Shift1/1 -> Minus/1

== system HANcoder_E407_TTA_Controller_v2/HANcoder STM32 Target - E407-STM32 algorithm/Global Ticks Increment/CAN Management/Matrix Cycle Manager/Subsystem/controller basic cycle 1/COMP Task - Rx_Set_Values_Check/Update Msg buffer/Set Values Update/uint8_2float1 ==
  precision : Inport
  value : Inport  Port=2
  Bit Shift : hdlsllib/Logic and Bit Operations/Bit Shift  mode=Shift Right Logical  N=7
      settings: SourceProductName=HDL Coder  SourceProductBaseCode=HD
  Bit Shift1 : hdlsllib/Logic and Bit Operations/Bit Shift  mode=Shift Left Logical  N=7
      settings: SourceProductName=HDL Coder  SourceProductBaseCode=HD
  Cast1 : DataTypeConversion  OutDataTypeStr=double
  Constant1 : Constant  Value=2
  Constant2 : Constant  Value=2
  Divide : Product  Inputs=*/
  Fix1 : Rounding  Operator=fix
  Gain : Gain  Gain=-1
  Gain1 : Gain  Gain=-1
  Minus : Sum  Inputs=-+
  Minus1 : Sum  Inputs=+-
  Minus2 : Sum
  Multiply : Product
  Multiply1 : Product
  Power : Math  Priority=5  Operator=pow  SaturateOnIntegerOverflow=on
  Power1 : Math  Priority=5  Operator=pow  SaturateOnIntegerOverflow=on
  Switch : Switch  Criteria=u2 > Threshold
  decoded : Outport
  wires:
  Bit Shift1/1 -> Minus/1
  [prec_pow] -> Multiply1/2
  [prec_pow] -> Divide/2
  Power1/1 -> [prec_pow]
  Constant2/1 -> Power1/1
  precision/1 -> [precision], Power1/2
  Cast1/1 -> Minus/2
  Divide/1 -> Fix1/1
  Switch/1 -> decoded/1
  Gain1/1 -> Switch/1
  Minus2/1 -> Switch/3, Gain1/1
  Multiply/1 -> Minus2/1
  [precision] -> Gain/1
  Power/1 -> Multiply/2
  Gain/1 -> Power/2
  Constant1/1 -> Power/1
  Minus1/1 -> Multiply/1
  Multiply1/1 -> Minus1/2
  Fix1/1 -> Multiply1/1, Minus2/2
  Minus/1 -> Minus1/1, Divide/1
  value/1 -> Bit Shift/1, Cast1/1
  Bit Shift/1 -> Switch/2, Bit Shift1/1

== system HANcoder_E407_TTA_Controller_v2/HANcoder STM32 Target - E407-STM32 algorithm/Global Ticks Increment/CAN Management/Matrix Cycle Manager/Subsystem/controller basic cycle 1/COMP Task - Rx_Set_Values_Check/Update Msg buffer/Set Values Update/uint8_2float2 ==
  precision : Inport
  value : Inport  Port=2
  Bit Shift : hdlsllib/Logic and Bit Operations/Bit Shift  mode=Shift Right Logical  N=7
      settings: SourceProductName=HDL Coder  SourceProductBaseCode=HD
  Bit Shift1 : hdlsllib/Logic and Bit Operations/Bit Shift  mode=Shift Left Logical  N=7
      settings: SourceProductName=HDL Coder  SourceProductBaseCode=HD
  Cast1 : DataTypeConversion  OutDataTypeStr=double
  Constant1 : Constant  Value=2
  Constant2 : Constant  Value=2
  Divide : Product  Inputs=*/
  Fix1 : Rounding  Operator=fix
  Gain : Gain  Gain=-1
  Gain1 : Gain  Gain=-1
  Minus : Sum  Inputs=-+
  Minus1 : Sum  Inputs=+-
  Minus2 : Sum
  Multiply : Product
  Multiply1 : Product
  Power : Math  Priority=5  Operator=pow  SaturateOnIntegerOverflow=on
  Power1 : Math  Priority=5  Operator=pow  SaturateOnIntegerOverflow=on
  Switch : Switch  Criteria=u2 > Threshold
  decoded : Outport
  wires:
  Bit Shift/1 -> Bit Shift1/1, Switch/2
  value/1 -> Cast1/1, Bit Shift/1
  Minus/1 -> Divide/1, Minus1/1
  Fix1/1 -> Minus2/2, Multiply1/1
  Multiply1/1 -> Minus1/2
  Minus1/1 -> Multiply/1
  Constant1/1 -> Power/1
  Gain/1 -> Power/2
  Power/1 -> Multiply/2
  [precision] -> Gain/1
  Multiply/1 -> Minus2/1
  Minus2/1 -> Gain1/1, Switch/3
  Gain1/1 -> Switch/1
  Switch/1 -> decoded/1
  Divide/1 -> Fix1/1
  Cast1/1 -> Minus/2
  precision/1 -> Power1/2, [precision]
  Constant2/1 -> Power1/1
  Power1/1 -> [prec_pow]
  [prec_pow] -> Divide/2
  [prec_pow] -> Multiply1/2
  Bit Shift1/1 -> Minus/1

== system HANcoder_E407_TTA_Controller_v2/HANcoder STM32 Target - E407-STM32 algorithm/Global Ticks Increment/CAN Management/Matrix Cycle Manager/Subsystem/controller basic cycle 1/COMP Task - Sync bc1 check/Process_Messages/Demux message CAN1 and check coherence/Subsystem ==
  Msg_Temporal_Data : Inport
  Bit Shift : hdlsllib/Logic and Bit Operations/Bit Shift  mode=Shift Right Logical  N=7
      settings: SourceProductName=HDL Coder  SourceProductBaseCode=HD
  Bit Shift1 : hdlsllib/Logic and Bit Operations/Bit Shift  mode=Shift Right Logical  N=5
      settings: SourceProductName=HDL Coder  SourceProductBaseCode=HD
  Bit Shift2 : hdlsllib/Logic and Bit Operations/Bit Shift  mode=Shift Right Logical  N=4
      settings: SourceProductName=HDL Coder  SourceProductBaseCode=HD
  Bit Shift3 : hdlsllib/Logic and Bit Operations/Bit Shift  mode=Shift Left Logical  N=1
      settings: SourceProductName=HDL Coder  SourceProductBaseCode=HD
  Bit Shift4 : hdlsllib/Logic and Bit Operations/Bit Shift  mode=Shift Left Logical  N=4
      settings: SourceProductName=HDL Coder  SourceProductBaseCode=HD
  basic_cycle : Outport
  msg_count : Outport  Port=2
  board_id : Outport  Port=3
  wires:
  Bit Shift4/1 -> Bit Shift2/1
  Bit Shift1/1 -> msg_count/1
  Bit Shift3/1 -> Bit Shift1/1
  Msg_Temporal_Data/1 -> Bit Shift4/1, Bit Shift/1, Bit Shift3/1
  Bit Shift/1 -> basic_cycle/1
  Bit Shift2/1 -> board_id/1

== system HANcoder_E407_TTA_Controller_v2/HANcoder STM32 Target - E407-STM32 algorithm/Global Ticks Increment/CAN Management/Matrix Cycle Manager/Subsystem/controller basic cycle 1/COMP Task - Sync bc1 check/Process_Messages/Demux message CAN1 and check coherence/msg_count>2_DEBUG ==
  note: If this board received during this COMM a message
      | with a count greater than 1, it means the first message
      | sent was missed, but at least one later msg reached
      | this board.
  msg_c : Inport
  Constant : Constant
  Constant1 : Constant
  Data Store Read : DataStoreRead  DataStoreName=msg_count_DEBUG
  Data Store Read1 : DataStoreRead  DataStoreName=msg_count_DEBUG
  Data Store Write : DataStoreWrite  DataStoreName=msg_count_DEBUG
  GreaterThan : RelationalOperator  Operator=>  OutDataTypeStr=boolean  RndMeth=Simplest
  Plus : Sum
  Switch : Switch  Criteria=u2 > Threshold
  wires:
  msg_c/1 -> GreaterThan/1
  Data Store Read/1 -> Switch/3
  Plus/1 -> Switch/1
  Data Store Read1/1 -> Plus/1
  Constant/1 -> Plus/2
  Switch/1 -> Data Store Write/1
  GreaterThan/1 -> Switch/2
  Constant1/1 -> GreaterThan/2

== system HANcoder_E407_TTA_Controller_v2/HANcoder STM32 Target - E407-STM32 algorithm/Global Ticks Increment/CAN Management/Matrix Cycle Manager/Subsystem/controller basic cycle 1/COMP Task - Sync bc1 check/Process_Messages/Demux message CAN1 and check coherence1/Subsystem ==
  Msg_Temporal_Data : Inport
  Bit Shift : hdlsllib/Logic and Bit Operations/Bit Shift  mode=Shift Right Logical  N=7
      settings: SourceProductName=HDL Coder  SourceProductBaseCode=HD
  Bit Shift1 : hdlsllib/Logic and Bit Operations/Bit Shift  mode=Shift Right Logical  N=5
      settings: SourceProductName=HDL Coder  SourceProductBaseCode=HD
  Bit Shift2 : hdlsllib/Logic and Bit Operations/Bit Shift  mode=Shift Right Logical  N=4
      settings: SourceProductName=HDL Coder  SourceProductBaseCode=HD
  Bit Shift3 : hdlsllib/Logic and Bit Operations/Bit Shift  mode=Shift Left Logical  N=1
      settings: SourceProductName=HDL Coder  SourceProductBaseCode=HD
  Bit Shift4 : hdlsllib/Logic and Bit Operations/Bit Shift  mode=Shift Left Logical  N=4
      settings: SourceProductName=HDL Coder  SourceProductBaseCode=HD
  basic_cycle : Outport
  msg_count : Outport  Port=2
  board_id : Outport  Port=3
  wires:
  Bit Shift/1 -> basic_cycle/1
  Msg_Temporal_Data/1 -> Bit Shift4/1, Bit Shift/1, Bit Shift3/1
  Bit Shift1/1 -> msg_count/1
  Bit Shift2/1 -> board_id/1
  Bit Shift3/1 -> Bit Shift1/1
  Bit Shift4/1 -> Bit Shift2/1

== system HANcoder_E407_TTA_Controller_v2/HANcoder STM32 Target - E407-STM32 algorithm/Global Ticks Increment/CAN Management/Matrix Cycle Manager/Subsystem/controller basic cycle 1/COMP Task - Sync bc1 check/Process_Messages/Demux message CAN1 and check coherence1/msg_count>2_DEBUG ==
  note: If this board received during this COMM a message
      | with a count greater than 1, it means the first message
      | sent was missed, but at least one later msg reached
      | this board.
  msg_c : Inport
  Constant : Constant
  Constant1 : Constant
  Data Store Read : DataStoreRead  DataStoreName=msg_count_DEBUG
  Data Store Read1 : DataStoreRead  DataStoreName=msg_count_DEBUG
  Data Store Write : DataStoreWrite  DataStoreName=msg_count_DEBUG
  GreaterThan : RelationalOperator  Operator=>  OutDataTypeStr=boolean  RndMeth=Simplest
  Plus : Sum
  Switch : Switch  Criteria=u2 > Threshold
  wires:
  msg_c/1 -> GreaterThan/1
  Data Store Read/1 -> Switch/3
  Plus/1 -> Switch/1
  Data Store Read1/1 -> Plus/1
  Constant/1 -> Plus/2
  Switch/1 -> Data Store Write/1
  GreaterThan/1 -> Switch/2
  Constant1/1 -> GreaterThan/2

== system HANcoder_E407_TTA_Controller_v2/HANcoder STM32 Target - E407-STM32 algorithm/Global Ticks Increment/CAN Management/Matrix Cycle Manager/Subsystem/controller basic cycle 0/COMM Task - Sync bc 0/Transmission subtasks/Check msg transmission CAN1/TX buffer update CAN1/Msg_Data_Encoder ==
  basic_cycle : Inport
  tx_counter : Inport  Port=2
  board_number : Inport  Port=3
  Bit Shift : hdlsllib/Logic and Bit Operations/Bit Shift  mode=Shift Left Logical  N=4
      settings: SourceProductName=HDL Coder  SourceProductBaseCode=HD
  Bit Shift1 : hdlsllib/Logic and Bit Operations/Bit Shift  mode=Shift Left Logical  N=7
      settings: SourceProductName=HDL Coder  SourceProductBaseCode=HD
  Minus : Sum  Inputs=3
  encoded_msg : Outport
  wires:
  basic_cycle/1 -> Bit Shift1/1
  Minus/1 -> encoded_msg/1
  tx_counter/1 -> Bit Shift/1
  Bit Shift1/1 -> Minus/1
  Bit Shift/1 -> Minus/2
  board_number/1 -> Minus/3

== system HANcoder_E407_TTA_Controller_v2/HANcoder STM32 Target - E407-STM32 algorithm/Global Ticks Increment/CAN Management/Matrix Cycle Manager/Subsystem/controller basic cycle 0/COMM Task - Sync bc 0/Transmission subtasks/Check msg transmission CAN2/TX buffer update CAN2/Msg_Data_Encoder ==
  basic_cycle : Inport
  tx_counter : Inport  Port=2
  verif_value : Inport  Port=3
  Bit Shift : hdlsllib/Logic and Bit Operations/Bit Shift  mode=Shift Left Logical  N=4
      settings: SourceProductName=HDL Coder  SourceProductBaseCode=HD
  Bit Shift1 : hdlsllib/Logic and Bit Operations/Bit Shift  mode=Shift Left Logical  N=7
      settings: SourceProductName=HDL Coder  SourceProductBaseCode=HD
  Minus : Sum  Inputs=3
  encoded_msg : Outport
  wires:
  basic_cycle/1 -> Bit Shift1/1
  Minus/1 -> encoded_msg/1
  tx_counter/1 -> Bit Shift/1
  Bit Shift1/1 -> Minus/1
  Bit Shift/1 -> Minus/2
  verif_value/1 -> Minus/3

== system HANcoder_E407_TTA_Controller_v2/HANcoder STM32 Target - E407-STM32 algorithm/Global Ticks Increment/CAN Management/Matrix Cycle Manager/Subsystem/controller basic cycle 0/COMM Task - Vote1/Transmission subtasks/Check msg transmission CAN1/TX buffer update CAN1/Msg_Data_Encoder ==
  basic_cycle : Inport
  tx_counter : Inport  Port=2
  board_number : Inport  Port=3
  Bit Shift : hdlsllib/Logic and Bit Operations/Bit Shift  mode=Shift Left Logical  N=4
      settings: SourceProductName=HDL Coder  SourceProductBaseCode=HD
  Bit Shift1 : hdlsllib/Logic and Bit Operations/Bit Shift  mode=Shift Left Logical  N=7
      settings: SourceProductName=HDL Coder  SourceProductBaseCode=HD
  Minus : Sum  Inputs=3
  encoded_msg : Outport
  wires:
  basic_cycle/1 -> Bit Shift1/1
  Minus/1 -> encoded_msg/1
  tx_counter/1 -> Bit Shift/1
  Bit Shift1/1 -> Minus/1
  Bit Shift/1 -> Minus/2
  board_number/1 -> Minus/3

== system HANcoder_E407_TTA_Controller_v2/HANcoder STM32 Target - E407-STM32 algorithm/Global Ticks Increment/CAN Management/Matrix Cycle Manager/Subsystem/controller basic cycle 0/COMM Task - Vote1/Transmission subtasks/Check msg transmission CAN2/TX buffer update CAN2/Msg_Data_Encoder ==
  basic_cycle : Inport
  tx_counter : Inport  Port=2
  verif_value : Inport  Port=3
  Bit Shift : hdlsllib/Logic and Bit Operations/Bit Shift  mode=Shift Left Logical  N=4
      settings: SourceProductName=HDL Coder  SourceProductBaseCode=HD
  Bit Shift1 : hdlsllib/Logic and Bit Operations/Bit Shift  mode=Shift Left Logical  N=7
      settings: SourceProductName=HDL Coder  SourceProductBaseCode=HD
  Minus : Sum  Inputs=3
  encoded_msg : Outport
  wires:
  basic_cycle/1 -> Bit Shift1/1
  Minus/1 -> encoded_msg/1
  tx_counter/1 -> Bit Shift/1
  Bit Shift1/1 -> Minus/1
  Bit Shift/1 -> Minus/2
  verif_value/1 -> Minus/3

== system HANcoder_E407_TTA_Controller_v2/HANcoder STM32 Target - E407-STM32 algorithm/Global Ticks Increment/CAN Management/Matrix Cycle Manager/Subsystem/controller basic cycle 0/COMM Task - Vote2/Transmission subtasks/Check msg transmission CAN1/TX buffer update CAN1/Msg_Data_Encoder ==
  basic_cycle : Inport
  tx_counter : Inport  Port=2
  board_number : Inport  Port=3
  Bit Shift : hdlsllib/Logic and Bit Operations/Bit Shift  mode=Shift Left Logical  N=4
      settings: SourceProductName=HDL Coder  SourceProductBaseCode=HD
  Bit Shift1 : hdlsllib/Logic and Bit Operations/Bit Shift  mode=Shift Left Logical  N=7
      settings: SourceProductName=HDL Coder  SourceProductBaseCode=HD
  Minus : Sum  Inputs=3
  encoded_msg : Outport
  wires:
  basic_cycle/1 -> Bit Shift1/1
  Minus/1 -> encoded_msg/1
  tx_counter/1 -> Bit Shift/1
  Bit Shift1/1 -> Minus/1
  Bit Shift/1 -> Minus/2
  board_number/1 -> Minus/3
